simulink model "atrias_boom_nmSt_kinSw_v4"  (R2015a)
settings: Solver=ode23t  StartTime=0.0  StopTime=t_end  FixedStep=0.001  MaxStep=1e-3  RelTol=1e-3
InitFcn:
  | addpath('../common/')
  | colors
StartFcn:
  | tic
StopFcn:
  | %stopscript
values from neighbouring files (symbols this model uses):
  dt_a_dTrunk_boom = 5    [main_1_nmSt_kinSw.m]    (also in main_2_nmSt_kinSw_v2.m; main_3_nmSt_kinSw_v3.m; main_4_nmSt_kinSw_v4.m)
  dt_fade_boomCtrl = 2    [main_1_nmSt_kinSw.m]    (also in main_2_nmSt_kinSw_v2.m; main_3_nmSt_kinSw_v3.m; main_4_nmSt_kinSw_v4.m)
  initial_boom_yaw = 15*pi/180    (= 0.261799387799)    [main_2_nmSt_kinSw_v2.m]    (also in main_3_nmSt_kinSw_v3.m; main_4_nmSt_kinSw_v4.m)
  kd_boom_roll_Ctrl = 0    [main_1_nmSt_kinSw - Copy.m]    (also in main_1_nmSt_kinSw.m; main_2_nmSt_kinSw_v2.m; main_3_nmSt_kinSw_v3.m; main_4_nmSt_kinSw_v4.m)
  kd_boom_yaw_Ctrl = 0.1*kp_boom_yaw_Ctrl    (= 100000000)    [main_1_nmSt_kinSw - Copy.m]    (also in main_1_nmSt_kinSw.m = 1000000000; main_2_nmSt_kinSw_v2.m = 10000000; main_3_nmSt_kinSw_v3.m = 10000000; main_4_nmSt_kinSw_v4.m = 10000000)
  kd_motor = 0.90*2*sqrt(3.75*kp_motor)    [main_1_nmSt_kinSw - Copy.m]
  kinSw_alpha_start = 100*pi/180    (= 1.74532925199)    [main_1_nmSt_kinSw - Copy.m]    (also in main_1_nmSt_kinSw.m = 1.91986217719; main_2_nmSt_kinSw_v2.m = 1.83259571459; main_3_nmSt_kinSw_v3.m = 1.83259571459; main_4_nmSt_kinSw_v4.m = 1.83259571459)
  kinSw_alpha_tgt = 80*pi/180    (= 1.3962634016)    [main_1_nmSt_kinSw - Copy.m]    (also in main_1_nmSt_kinSw.m = 1.2217304764; main_2_nmSt_kinSw_v2.m = 1.2217304764; main_3_nmSt_kinSw_v3.m = 1.2217304764; main_4_nmSt_kinSw_v4.m = 1.2217304764)
  kinSw_t_start = 1.5    [main_1_nmSt_kinSw - Copy.m]    (also in main_1_nmSt_kinSw.m; main_2_nmSt_kinSw_v2.m = 0.5; main_3_nmSt_kinSw_v3.m = 0.5; main_4_nmSt_kinSw_v4.m = 0.5)
  kp_boom_roll_Ctrl = 0    [main_1_nmSt_kinSw - Copy.m]    (also in main_1_nmSt_kinSw.m; main_2_nmSt_kinSw_v2.m; main_3_nmSt_kinSw_v3.m; main_4_nmSt_kinSw_v4.m)
  kp_boom_yaw_Ctrl = 1e9    (= 1000000000)    [main_1_nmSt_kinSw - Copy.m]    (also in main_1_nmSt_kinSw.m = 10000000000; main_2_nmSt_kinSw_v2.m = 100000000; main_3_nmSt_kinSw_v3.m = 100000000; main_4_nmSt_kinSw_v4.m = 100000000)
  kp_motor = 3000    [main_1_nmSt_kinSw - Copy.m]
  max_back_bar_angle = 262.4*pi/180    (= 4.57974395723)    [main_1_nmSt_kinSw - Copy.m]
  max_front_bar_angle = 194.8*pi/180    (= 3.39990138288)    [main_1_nmSt_kinSw - Copy.m]
  min_back_bar_angle = 165.0*pi/180    (= 2.87979326579)    [main_1_nmSt_kinSw - Copy.m]
  min_front_bar_angle = 98.0*pi/180    (= 1.71042266695)    [main_1_nmSt_kinSw - Copy.m]
  poser_LLegAlp = (initial_l_leg_angle -pi/2)*180/pi    (= 105)    [main_2_nmSt_kinSw_v2.m]    (also in main_3_nmSt_kinSw_v3.m; main_4_nmSt_kinSw_v4.m)
  poser_LLegLen = initial_l_leg_length    (= 0.88)    [main_2_nmSt_kinSw_v2.m]    (also in main_3_nmSt_kinSw_v3.m; main_4_nmSt_kinSw_v4.m)
  poser_RLegAlp = (initial_r_leg_angle -pi/2)*180/pi    (= 75)    [main_2_nmSt_kinSw_v2.m]    (also in main_3_nmSt_kinSw_v3.m; main_4_nmSt_kinSw_v4.m)
  poser_RLegLen = initial_r_leg_length    (= 0.9)    [main_2_nmSt_kinSw_v2.m]    (also in main_3_nmSt_kinSw_v3.m; main_4_nmSt_kinSw_v4.m)
  tEnd_boomCtrl = t_end    (= 20)    [main_1_nmSt_kinSw - Copy.m]    (also in main_1_nmSt_kinSw.m = 3; main_2_nmSt_kinSw_v2.m = 7.5; main_3_nmSt_kinSw_v3.m = 7.5; main_4_nmSt_kinSw_v4.m = 7.5)
  tStart_boomCtrl = 1    [main_1_nmSt_kinSw - Copy.m]    (also in main_1_nmSt_kinSw.m = 0; main_2_nmSt_kinSw_v2.m = 0.5; main_3_nmSt_kinSw_v3.m = 0.5; main_4_nmSt_kinSw_v4.m = 0.5)
  tune_kinSw_alpha_start = kinSw_alpha_start*180/pi    (= 105)    [main_2_nmSt_kinSw_v2.m]    (also in main_3_nmSt_kinSw_v3.m; main_4_nmSt_kinSw_v4.m)
  tune_kinSw_alpha_tgt = kinSw_alpha_tgt*180/pi    (= 70)    [main_2_nmSt_kinSw_v2.m]    (also in main_3_nmSt_kinSw_v3.m; main_4_nmSt_kinSw_v4.m)
  tune_kinSw_gClr_tgt = kinSw_gClr    (= 0.15)    [main_4_nmSt_kinSw_v4.m]
  tune_kinSw_gH_tgt = kinSw_gH_tgt    (= -0.01)    [main_4_nmSt_kinSw_v4.m]
  tune_M1_G = St_FGain_VAS*FmaxVAS    [main_2_nmSt_kinSw_v2.m]    (also in main_3_nmSt_kinSw_v3.m; main_4_nmSt_kinSw_v4.m)
  tune_M3_0 = CtrlPar_theta0*180/pi    [main_2_nmSt_kinSw_v2.m]    (also in main_3_nmSt_kinSw_v3.m; main_4_nmSt_kinSw_v4.m)
  tune_M3_D = St_GainDTh_HFL    [main_2_nmSt_kinSw_v2.m]    (also in main_3_nmSt_kinSw_v3.m; main_4_nmSt_kinSw_v4.m)
  tune_M3_P = St_GainTh_HFL    [main_2_nmSt_kinSw_v2.m]    (also in main_3_nmSt_kinSw_v3.m; main_4_nmSt_kinSw_v4.m)
  tune_M4_G = 1    [main_3_nmSt_kinSw_v3.m]    (also in main_4_nmSt_kinSw_v4.m)
  v_dTrunk_boom = 1.3    [main_1_nmSt_kinSw.m]    (also in main_2_nmSt_kinSw_v2.m; main_3_nmSt_kinSw_v3.m; main_4_nmSt_kinSw_v4.m)
undefined symbols (not defined in the file or in its folder): A1_notch_f1, A2_notch_f1, A_lpf_dtau, A_lpf_velocity, ankle_stiffness, B1_lpf_dtau, B1_lpf_velocity, B1_notch_f1, B2_lpf_dtau, B2_lpf_velocity, B2_notch_f1, b_hmotor, b_leg_spring, b_rotor, base_color_d, boom_color_d, boom_mount_to_center_diagonal, breakaway_friction, c_jointstop, contactThr, coulomb_friction, d_com, delta_phi_max, delta_phi_max_buffer, delta_phi_max_dropoff, delta_phi_min, fblink_color_d, floor_color_d, FmaxBFSH, FmaxGLU, FmaxHAM, FmaxHFL, FmaxRF, FmaxVAS, foot_color_d, FPCtrlPar, friction_linear_zone, g, gain_nodes_sea_torque, HIP_MTR_MAX_CONT_TORQUE, HIP_MTR_MAX_TORQUE, hshaft_color_d, initial_boom_pitch, initial_boom_roll, initial_hip_roll, initial_winch_angle, j_motor, k_gn, k_gt, k_leg_spring, K_notch_f1, k_phi, k_sea, Kb_leg, kd_lateral, kd_shin_max, kd_shin_min, kd_splay_max, kd_splay_min, kd_thigh_max ... (+186)
libraries: sm_lib x210, nesl_utility x140, simulink x65, simulink_extras x32, fl_lib x16, mblibv1 x2, commnoisgen2 x1
(part 16 of 17)

== system atrias_boom_nmSt_kinSw_v4/Control/Behavior Control/Virtual Neuromuscular Control/Muscle Layer/VAS1/BE force-length relation ==
  note: Buffer Elasticity BE
  lce [lopt] : Inport
  Constant1 : Constant  Value=1-mtu_w
  Math Function : Math  Operator=square  SaturateOnIntegerOverflow=on
  Mux1 : Mux  Inputs=2
  Sum4 : Sum  Inputs=|+-  SaturateOnIntegerOverflow=on  InputSameDT=on  OutDataTypeStr=Inherit: Same as first input
  force above slack length : Fcn  Expr=u(2)*(u(1)<0)
  reference strain [lslack] : Constant  Value=mtu_w/2
  relative strain : Product  Inputs=*/
  fbe [Fmax] : Outport
  wires:
  lce [lopt]/1 -> Sum4/1
  Mux1/1 -> force above slack length/1
  force above slack length/1 -> fbe [Fmax]/1
  Math Function/1 -> Mux1/2
  relative strain/1 -> Math Function/1
  reference strain [lslack]/1 -> relative strain/2
  Sum4/1 -> relative strain/1, Mux1/1
  Constant1/1 -> Sum4/2

== system atrias_boom_nmSt_kinSw_v4/Control/Behavior Control/Virtual Neuromuscular Control/Muscle Layer/VAS1/CE force-length relation ==
  note: CE Force-Length Relationship
  lce [lopt] : Inport
  Abs : Abs
  Constant1 : Constant
  Constant2 : Constant  Value=3
  Gain : Gain  Gain=log(mtu_c)
  Math Function : Math  SaturateOnIntegerOverflow=on
  Math Function1 : Math  Operator=pow  SaturateOnIntegerOverflow=on
  Sum4 : Sum  Inputs=|+-  SaturateOnIntegerOverflow=on  InputSameDT=on  OutDataTypeStr=Inherit: Same as first input
  normalized position : Product  Inputs=*/
  relative width : Constant  Value=mtu_w
  fce [Fmax] : Outport
  wires:
  lce [lopt]/1 -> Sum4/1
  relative width/1 -> normalized position/2
  Constant1/1 -> Sum4/2
  Sum4/1 -> Abs/1
  Abs/1 -> normalized position/1
  normalized position/1 -> Math Function1/1
  Constant2/1 -> Math Function1/2
  Math Function1/1 -> Gain/1
  Gain/1 -> Math Function/1
  Math Function/1 -> fce [Fmax]/1

== system atrias_boom_nmSt_kinSw_v4/Control/Behavior Control/Virtual Neuromuscular Control/Muscle Layer/VAS1/CE inverse force-velocity relation ==
  note: CE Inverse Force-Velocity Relationship
  Fv[Fmax] : Inport
  1 : Product  Inputs=/*
  Constant{1,3..4,8} (4 alike) : Constant
  Constant2 : Constant  Value=mtu_N
  Constant5 : Constant  Value=mtu_N
  Curvature : Gain  Gain=mtu_K  SaturateOnIntegerOverflow=on  OutDataTypeStr=Inherit: Same as input  ParamDataTypeStr=Inherit: Same as input
  Curvature1 : Gain  Gain=7.56*mtu_K  SaturateOnIntegerOverflow=on  OutDataTypeStr=Inherit: Same as input  ParamDataTypeStr=Inherit: Same as input
  Mux : Mux  Inputs=2
  Mux1 : Mux  Inputs=3
  Mux2 : Mux  Inputs=3
  Slope : Gain  Gain=1e-2  SaturateOnIntegerOverflow=on  OutDataTypeStr=Inherit: Same as input  ParamDataTypeStr=Inherit: Same as input
  Sum1 : Sum  Inputs=|++  SaturateOnIntegerOverflow=on  InputSameDT=on  OutDataTypeStr=Inherit: Same as first input
  Sum2 : Sum  SaturateOnIntegerOverflow=on  InputSameDT=on  OutDataTypeStr=Inherit: Same as first input
  Sum3 : Sum  Inputs=++|  SaturateOnIntegerOverflow=on  InputSameDT=on  OutDataTypeStr=Inherit: Same as first input
  Sum4 : Sum  Inputs=|+-  SaturateOnIntegerOverflow=on  InputSameDT=on  OutDataTypeStr=Inherit: Same as first input
  Sum5 : Sum  Inputs=|-+  SaturateOnIntegerOverflow=on  InputSameDT=on  OutDataTypeStr=Inherit: Same as first input
  Sum6 : Sum  Inputs=-+|  SaturateOnIntegerOverflow=on  InputSameDT=on  OutDataTypeStr=Inherit: Same as first input
  Sum7 : Sum  Inputs=|++  SaturateOnIntegerOverflow=on  InputSameDT=on  OutDataTypeStr=Inherit: Same as first input
  Sum8 : Sum  Inputs=+-|  SaturateOnIntegerOverflow=on  InputSameDT=on  OutDataTypeStr=Inherit: Same as first input
  Sum9 : Sum  SaturateOnIntegerOverflow=on  InputSameDT=on  OutDataTypeStr=Inherit: Same as first input
  concentric branch : Fcn  Expr=u(1) * (u(2)<=1)
  excentric branch : Fcn  Expr=u(2) * (u(1)>1)*(u(1)<=u(3))
  excentric overshoot : Fcn  Expr=u(3) * (u(2)>u(1))
  v_concentric : Product  Inputs=*/
  v_excentric <N : Product  Inputs=*/
  v[vmax] : Outport
  wires:
  Curvature/1 -> Sum3/2
  Constant1/1 -> Sum4/2, Sum3/1
  Sum4/1 -> v_concentric/1
  Sum3/1 -> v_concentric/2
  1/1 -> Sum7/1, Curvature1/1
  Constant4/1 -> Sum7/2, Sum8/1
  Curvature1/1 -> Sum8/2
  Sum8/1 -> v_excentric <N/2
  Sum7/1 -> v_excentric <N/1
  v_concentric/1 -> Mux/1
  Fv[Fmax]/1 -> Sum4/1, Curvature/1, Sum6/2, Mux/2, Mux1/1, Mux2/2
  Sum9/1 -> v[vmax]/1
  Sum2/1 -> Sum9/2
  excentric overshoot/1 -> Sum2/2
  Slope/1 -> Sum1/1
  Constant8/1 -> Sum1/2
  Sum6/1 -> 1/2, Slope/1
  Constant2/1 -> Sum6/1, Sum5/2
  Sum5/1 -> 1/1
  Constant3/1 -> Sum5/1
  Mux/1 -> concentric branch/1
  Mux1/1 -> excentric branch/1
  v_excentric <N/1 -> Mux1/2
  Mux2/1 -> excentric overshoot/1
  concentric branch/1 -> Sum9/1
  excentric branch/1 -> Sum2/1
  Constant5/1 -> Mux1/3, Mux2/1
  Sum1/1 -> Mux2/3

== system atrias_boom_nmSt_kinSw_v4/Control/Behavior Control/Virtual Neuromuscular Control/Muscle Layer/VAS1/PE force-length relation ==
  note: Parallel Elasticity PE
  lce [lopt] : Inport
  Constant3 : Constant
  Math Function2 : Math  Operator=square  SaturateOnIntegerOverflow=on
  Mux : Mux  Inputs=2
  Sum1 : Sum  Inputs=|+-  SaturateOnIntegerOverflow=on  InputSameDT=on  OutDataTypeStr=Inherit: Same as first input
  force above slack length : Fcn  Expr=u(2) * (u(1)>1)
  reference strain [lopt] : Constant  Value=mtu_w
  relative strain : Product  Inputs=*/
  fpe [Fmax] : Outport
  wires:
  Mux/1 -> force above slack length/1
  lce [lopt]/1 -> Mux/1, Sum1/1
  Constant3/1 -> Sum1/2
  Sum1/1 -> relative strain/1
  reference strain [lopt]/1 -> relative strain/2
  relative strain/1 -> Math Function2/1
  Math Function2/1 -> Mux/2
  force above slack length/1 -> fpe [Fmax]/1

== system atrias_boom_nmSt_kinSw_v4/Control/Behavior Control/Virtual Neuromuscular Control/Muscle Layer/VAS1/SE force-length relation ==
  note: SE Force-Length Relationship
  lse [lslack] : Inport
  Constant1 : Constant
  Math Function : Math  Operator=square  SaturateOnIntegerOverflow=on
  Mux : Mux  Inputs=2
  Sum4 : Sum  Inputs=|+-  SaturateOnIntegerOverflow=on  InputSameDT=on  OutDataTypeStr=Inherit: Same as first input
  force above slack length : Fcn  Expr=u(2)*(u(1)>1)
  reference strain [lslack] : Constant  Value=mtu_eref
  relative strain : Product  Inputs=*/
  fse [Fmax] : Outport
  wires:
  Mux/1 -> force above slack length/1
  force above slack length/1 -> fse [Fmax]/1
  Math Function/1 -> Mux/2
  lse [lslack]/1 -> Mux/1, Sum4/1
  relative strain/1 -> Math Function/1
  reference strain [lslack]/1 -> relative strain/2
  Sum4/1 -> relative strain/1
  Constant1/1 -> Sum4/2

== system atrias_boom_nmSt_kinSw_v4/Control/Behavior Control/Virtual Neuromuscular Control/Torque Distribution/mech limit avoidance1/PD Joint Limit ==
  L Mechanical Limit Avoidance Torque : Subsystem
  L scale desired torque : Subsystem
  Mux1 : Mux
  Mux2 : Mux
  R Mechanical Limit Avoidance Torque : Subsystem
  R scale desired torque : Subsystem
  tau_pd_hip_knee [Nm]x4 : Outport
  des_trq_scale x4 : Outport  Port=2
  tag scope: L_scale_hip=global, L_scale_knee=global, Ltau_pd_hip=global, Ltau_pd_knee=global, R_scale_hip=global, R_scale_knee=global, Rtau_pd_hip=global, Rtau_pd_knee=global
  wires:
  L scale desired torque/2(scale_knee) -> [L_scale_knee]
  L scale desired torque/1(scale_hip) -> [L_scale_hip]
  [Lphi_shin] -> L scale desired torque/2(phi_shin [rad])
  [Lphi_thigh] -> L scale desired torque/1(phi_thigh [rad])
  R Mechanical Limit Avoidance Torque/1(tau_pd_hip [Nm]) -> [Rtau_pd_hip]
  L Mechanical Limit Avoidance Torque/2(tau_pd_knee [Nm]) -> [Ltau_pd_knee]
  L Mechanical Limit Avoidance Torque/1(tau_pd_hip [Nm]) -> [Ltau_pd_hip]
  R Mechanical Limit Avoidance Torque/2(tau_pd_knee [Nm]) -> [Rtau_pd_knee]
  Mux2/1 -> tau_pd_hip_knee [Nm]x4/1
  [Rtau_pd_hip] -> Mux2/1
  [Rtau_pd_knee] -> Mux2/2
  [Ltau_pd_hip] -> Mux2/3
  [Ltau_pd_knee] -> Mux2/4
  Mux1/1 -> des_trq_scale x4/1
  [R_scale_hip] -> Mux1/1
  [R_scale_knee] -> Mux1/2
  [L_scale_hip] -> Mux1/3
  [L_scale_knee] -> Mux1/4
  R scale desired torque/2(scale_knee) -> [R_scale_knee]
  R scale desired torque/1(scale_hip) -> [R_scale_hip]
  [Rphi_shin] -> R scale desired torque/2(phi_shin [rad])
  [Rphi_thigh] -> R scale desired torque/1(phi_thigh [rad])
  [Rdphi_shin] -> R Mechanical Limit Avoidance Torque/4(dphi_shin [rad/s])
  [Rdphi_thigh] -> R Mechanical Limit Avoidance Torque/3(dphi_thigh [rad/s])
  [Rphi_shin] -> R Mechanical Limit Avoidance Torque/2(phi_shin [rad])
  [Rphi_thigh] -> R Mechanical Limit Avoidance Torque/1(phi_thigh [rad])
  [Ldphi_shin] -> L Mechanical Limit Avoidance Torque/4(dphi_shin [rad/s])
  [Ldphi_thigh] -> L Mechanical Limit Avoidance Torque/3(dphi_thigh [rad/s])
  [Lphi_shin] -> L Mechanical Limit Avoidance Torque/2(phi_shin [rad])
  [Lphi_thigh] -> L Mechanical Limit Avoidance Torque/1(phi_thigh [rad])

== system atrias_boom_nmSt_kinSw_v4/Control/Behavior Control/Virtual Neuromuscular Control/Torque Distribution/mech limit avoidance1/PD Joint Limit1 ==
  Demux : Demux
  Lechanical Limit Avoidance Torques : Subsystem
  Mux1 : Mux
  R Mechanical Limit Avoidance Torque : Subsystem
  R scale desired torque : Subsystem
  R scale desired torque1 : Subsystem
  to hip_knee : MATLAB Function  TreatAsAtomicUnit=on
  tau_pd_hip_knee [Nm]x4 : Outport
  des_trq_scale x4 : Outport  Port=2
  tag scope: L_scale_hip=global, L_scale_knee=global, Ltau_pd_back=global, Ltau_pd_front=global, Ltau_pd_hip=global, Ltau_pd_knee=global, R_scale_hip=global, R_scale_knee=global, Rtau_pd_back=global, Rtau_pd_front=global, Rtau_pd_hip=global, Rtau_pd_knee=global
  wires:
  [Lphi_thigh] -> Lechanical Limit Avoidance Torques/1(phi_thigh [rad])
  [Lphi_shin] -> Lechanical Limit Avoidance Torques/2(phi_shin [rad])
  [Ldphi_thigh] -> Lechanical Limit Avoidance Torques/3(dphi_thigh [rad/s])
  [Ldphi_shin] -> Lechanical Limit Avoidance Torques/4(dphi_shin [rad/s])
  Lechanical Limit Avoidance Torques/1(tau_pd_back [Nm]) -> [Ltau_pd_back]
  Lechanical Limit Avoidance Torques/2(tau_pd_front [Nm]) -> [Ltau_pd_front]
  [Rphi_thigh] -> R Mechanical Limit Avoidance Torque/1(phi_thigh [rad])
  [Rphi_shin] -> R Mechanical Limit Avoidance Torque/2(phi_shin [rad])
  [Rdphi_thigh] -> R Mechanical Limit Avoidance Torque/3(dphi_thigh [rad/s])
  [Rdphi_shin] -> R Mechanical Limit Avoidance Torque/4(dphi_shin [rad/s])
  R Mechanical Limit Avoidance Torque/1(tau_pd_back [Nm]) -> [Rtau_pd_back]
  R Mechanical Limit Avoidance Torque/2(tau_pd_front [Nm]) -> [Rtau_pd_front]
  [Rphi_thigh] -> R scale desired torque/1(phi_thigh [rad])
  [Rphi_shin] -> R scale desired torque/2(phi_shin [rad])
  R scale desired torque/1(scale_hip) -> [R_scale_hip]
  R scale desired torque/2(scale_knee) -> [R_scale_knee]
  [k_R] -> to hip_knee/5(kR)
  [k_L] -> to hip_knee/6(kL)
  [Ltau_pd_front] -> to hip_knee/4(Ltau_front)
  [Ltau_pd_back] -> to hip_knee/3(Ltau_back)
  [Rtau_pd_front] -> to hip_knee/2(Rtau_front)
  [Rtau_pd_back] -> to hip_knee/1(Rtau_back)
  to hip_knee/1(tau_pd_hip_knee) -> tau_pd_hip_knee [Nm]x4/1, Demux/1
  [k_R] -> R scale desired torque/3(k)
  [Lphi_thigh] -> R scale desired torque1/1(phi_thigh [rad])
  [Lphi_shin] -> R scale desired torque1/2(phi_shin [rad])
  R scale desired torque1/1(scale_hip) -> [L_scale_hip]
  R scale desired torque1/2(scale_knee) -> [L_scale_knee]
  [k_L] -> R scale desired torque1/3(k)
  [L_scale_knee] -> Mux1/4
  [L_scale_hip] -> Mux1/3
  [R_scale_knee] -> Mux1/2
  [R_scale_hip] -> Mux1/1
  Mux1/1 -> des_trq_scale x4/1
  Demux/1 -> [Rtau_pd_hip]
  Demux/2 -> [Rtau_pd_knee]
  Demux/3 -> [Ltau_pd_hip]
  Demux/4 -> [Ltau_pd_knee]

== system atrias_boom_nmSt_kinSw_v4/Mechanical System Layer/Ground Contact Models/L Back Ground Contact/3D Contact/Kinetic Friction Model/Vector Norm ==
  vec : Inport
  Sqrt : Sqrt  OutputSignalType=real  AlgorithmType=Newton-Raphson  SaturateOnIntegerOverflow=on
  Squares : Math  Operator=square  OutputSignalType=real  SaturateOnIntegerOverflow=on
  Sum of Elements : Sum  Inputs=+
  norm : Outport
  wires:
  vec/1 -> Squares/1
  Sqrt/1 -> norm/1
  Sum of Elements/1 -> Sqrt/1
  Squares/1 -> Sum of Elements/1

== system atrias_boom_nmSt_kinSw_v4/Mechanical System Layer/Ground Contact Models/L Back Ground Contact/3D Contact/Static Friction Model/Vector Norm ==
  vec : Inport
  Sqrt : Sqrt  OutputSignalType=real  AlgorithmType=Newton-Raphson  SaturateOnIntegerOverflow=on
  Squares : Math  Operator=square  OutputSignalType=real  SaturateOnIntegerOverflow=on
  Sum of Elements : Sum  Inputs=+
  norm : Outport
  wires:
  vec/1 -> Squares/1
  Sqrt/1 -> norm/1
  Sum of Elements/1 -> Sqrt/1
  Squares/1 -> Sum of Elements/1

== system atrias_boom_nmSt_kinSw_v4/Mechanical System Layer/Ground Contact Models/L Front Ground Contact/3D Contact/Kinetic Friction Model/Vector Norm ==
  vec : Inport
  Sqrt : Sqrt  OutputSignalType=real  AlgorithmType=Newton-Raphson  SaturateOnIntegerOverflow=on
  Squares : Math  Operator=square  OutputSignalType=real  SaturateOnIntegerOverflow=on
  Sum of Elements : Sum  Inputs=+
  norm : Outport
  wires:
  vec/1 -> Squares/1
  Sqrt/1 -> norm/1
  Sum of Elements/1 -> Sqrt/1
  Squares/1 -> Sum of Elements/1

== system atrias_boom_nmSt_kinSw_v4/Mechanical System Layer/Ground Contact Models/L Front Ground Contact/3D Contact/Static Friction Model/Vector Norm ==
  vec : Inport
  Sqrt : Sqrt  OutputSignalType=real  AlgorithmType=Newton-Raphson  SaturateOnIntegerOverflow=on
  Squares : Math  Operator=square  OutputSignalType=real  SaturateOnIntegerOverflow=on
  Sum of Elements : Sum  Inputs=+
  norm : Outport
  wires:
  vec/1 -> Squares/1
  Sqrt/1 -> norm/1
  Sum of Elements/1 -> Sqrt/1
  Squares/1 -> Sum of Elements/1

== system atrias_boom_nmSt_kinSw_v4/Mechanical System Layer/Ground Contact Models/R Back Ground Contact/3D Contact/Kinetic Friction Model/Vector Norm ==
  vec : Inport
  Sqrt : Sqrt  OutputSignalType=real  AlgorithmType=Newton-Raphson  SaturateOnIntegerOverflow=on
  Squares : Math  Operator=square  OutputSignalType=real  SaturateOnIntegerOverflow=on
  Sum of Elements : Sum  Inputs=+
  norm : Outport
  wires:
  vec/1 -> Squares/1
  Sqrt/1 -> norm/1
  Sum of Elements/1 -> Sqrt/1
  Squares/1 -> Sum of Elements/1

== system atrias_boom_nmSt_kinSw_v4/Mechanical System Layer/Ground Contact Models/R Back Ground Contact/3D Contact/Static Friction Model/Vector Norm ==
  vec : Inport
  Sqrt : Sqrt  OutputSignalType=real  AlgorithmType=Newton-Raphson  SaturateOnIntegerOverflow=on
  Squares : Math  Operator=square  OutputSignalType=real  SaturateOnIntegerOverflow=on
  Sum of Elements : Sum  Inputs=+
  norm : Outport
  wires:
  vec/1 -> Squares/1
  Sqrt/1 -> norm/1
  Sum of Elements/1 -> Sqrt/1
  Squares/1 -> Sum of Elements/1

== system atrias_boom_nmSt_kinSw_v4/Mechanical System Layer/Ground Contact Models/R Front Ground Contact/3D Contact/Kinetic Friction Model/Vector Norm ==
  vec : Inport
  Sqrt : Sqrt  OutputSignalType=real  AlgorithmType=Newton-Raphson  SaturateOnIntegerOverflow=on
  Squares : Math  Operator=square  OutputSignalType=real  SaturateOnIntegerOverflow=on
  Sum of Elements : Sum  Inputs=+
  norm : Outport
  wires:
  vec/1 -> Squares/1
  Sqrt/1 -> norm/1
  Sum of Elements/1 -> Sqrt/1
  Squares/1 -> Sum of Elements/1

== system atrias_boom_nmSt_kinSw_v4/Mechanical System Layer/Ground Contact Models/R Front Ground Contact/3D Contact/Static Friction Model/Vector Norm ==
  vec : Inport
  Sqrt : Sqrt  OutputSignalType=real  AlgorithmType=Newton-Raphson  SaturateOnIntegerOverflow=on
  Squares : Math  Operator=square  OutputSignalType=real  SaturateOnIntegerOverflow=on
  Sum of Elements : Sum  Inputs=+
  norm : Outport
  wires:
  vec/1 -> Squares/1
  Sqrt/1 -> norm/1
  Sum of Elements/1 -> Sqrt/1
  Squares/1 -> Sum of Elements/1

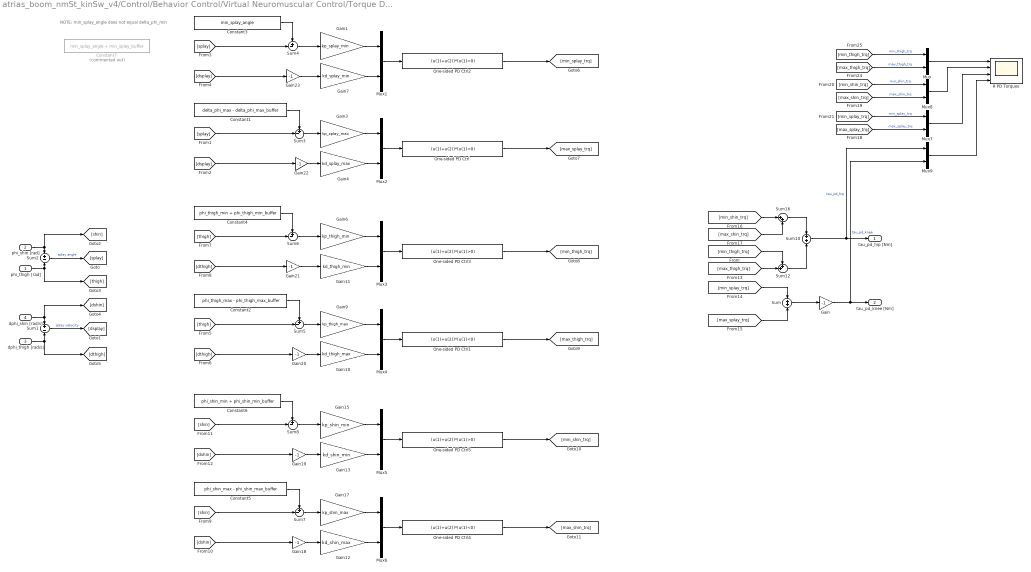
== system atrias_boom_nmSt_kinSw_v4/Control/Behavior Control/Virtual Neuromuscular Control/Torque Distribution/mech limit avoidance1/PD Joint Limit/L Mechanical Limit Avoidance Torque ==
  note: NOTE: min_splay_angle does not equal delta_phi_min
  phi_thigh [rad] : Inport
  phi_shin [rad] : Inport  Port=2
  dphi_thigh [rad/s] : Inport  Port=3
  dphi_shin [rad/s] : Inport  Port=4
  Constant1 : Constant  Value=delta_phi_max - delta_phi_max_buffer
  Constant2 : Constant  Value=phi_thigh_max - phi_thigh_max_buffer
  Constant3 : Constant  Value=min_splay_angle
  Constant4 : Constant  Value=phi_thigh_min + phi_thigh_min_buffer
  Constant5 : Constant  Value=phi_shin_max - phi_shin_max_buffer
  Constant6 : Constant  Value=phi_shin_min + phi_shin_min_buffer
  Constant7 : Constant  Commented=on  Value=min_splay_angle + min_splay_buffer
  Gain{,18..23} (7 alike) : Gain  Gain=-1
  Gain1 : Gain  Gain=kp_splay_min
  Gain10 : Gain  Gain=kd_thigh_max
  Gain11 : Gain  Gain=kd_thigh_min
  Gain12 : Gain  Gain=kd_shin_max
  Gain13 : Gain  Gain=kd_shin_min
  Gain15 : Gain  Gain=kp_shin_min
  Gain17 : Gain  Gain=kp_shin_max
  Gain3 : Gain  Gain=kp_splay_max
  Gain4 : Gain  Gain=kd_splay_max
  Gain6 : Gain  Gain=kp_thigh_min
  Gain7 : Gain  Gain=kd_splay_min
  Gain9 : Gain  Gain=kp_thigh_max
  Mux{,1..9} (10 alike) : Mux  Inputs=2
  One-sided PD Ctrl : Fcn  Expr=(u(1)+u(2))*(u(1)<0)
  One-sided PD Ctrl1 : Fcn  Expr=(u(1)+u(2))*(u(1)<0)
  One-sided PD Ctrl2 : Fcn  Expr=(u(1)+u(2))*(u(1)>0)
  One-sided PD Ctrl3 : Fcn  Expr=(u(1)+u(2))*(u(1)>0)
  One-sided PD Ctrl4 : Fcn  Expr=(u(1)+u(2))*(u(1)<0)
  One-sided PD Ctrl5 : Fcn  Expr=(u(1)+u(2))*(u(1)>0)
  R PD Torques : Scope  NumInputPorts=4
      settings: ShowLegends=on  TimeRange=2.5  YMin=-100~-5e+07~-1e+07~-5  YMax=100~1e+07~5e+07~5  SaveName=ScopeData5
  Sum : Sum
  Sum1 : Sum  Inputs=+-
  Sum10 : Sum
  Sum12 : Sum  Inputs=++|
  Sum16 : Sum  Inputs=|++
  Sum2 : Sum  Inputs=+-
  Sum{3..8} (6 alike) : Sum  Inputs=+-|
  tau_pd_hip [Nm] : Outport
  tau_pd_knee [Nm] : Outport  Port=2
  wires:
  One-sided PD Ctrl4/1 -> [max_shin_trq]
  One-sided PD Ctrl5/1 -> [min_shin_trq]
  One-sided PD Ctrl1/1 -> [max_thigh_trq]
  One-sided PD Ctrl3/1 -> [min_thigh_trq]
  One-sided PD Ctrl/1 -> [max_splay_trq]
  Gain23/1 -> Gain7/1
  Gain22/1 -> Gain4/1
  Gain21/1 -> Gain11/1
  Gain20/1 -> Gain10/1
  Gain19/1 -> Gain13/1
  Gain18/1 -> Gain12/1
  [max_splay_trq] -> Mux7/2  "max_splay_trq"
  [min_splay_trq] -> Mux7/1  "min_splay_trq"
  Mux7/1 -> R PD Torques/3
  Mux8/1 -> R PD Torques/2
  [max_shin_trq] -> Mux8/2  "max_shin_trq"
  [min_shin_trq] -> Mux8/1  "min_shin_trq"
  Mux/1 -> R PD Torques/1
  [max_thigh_trq] -> Mux/2  "max_thigh_trq"
  [min_thigh_trq] -> Mux/1  "min_thigh_trq"
  One-sided PD Ctrl2/1 -> [min_splay_trq]
  Mux6/1 -> One-sided PD Ctrl4/1
  Constant5/1 -> Sum7/1
  Sum7/1 -> Gain17/1
  Gain17/1 -> Mux6/1
  Gain12/1 -> Mux6/2
  [shin] -> Sum7/2
  [dshin] -> Gain18/1
  Mux5/1 -> One-sided PD Ctrl5/1
  Constant6/1 -> Sum8/1
  Sum8/1 -> Gain15/1
  Gain15/1 -> Mux5/1
  Gain13/1 -> Mux5/2
  [shin] -> Sum8/2
  [dshin] -> Gain19/1
  Mux4/1 -> One-sided PD Ctrl1/1
  Constant2/1 -> Sum5/1
  Sum5/1 -> Gain9/1
  Gain9/1 -> Mux4/1
  Gain10/1 -> Mux4/2
  [thigh] -> Sum5/2
  [dthigh] -> Gain20/1
  Mux3/1 -> One-sided PD Ctrl3/1
  Constant4/1 -> Sum6/1
  Sum6/1 -> Gain6/1
  Gain6/1 -> Mux3/1
  Gain11/1 -> Mux3/2
  [thigh] -> Sum6/2
  [dthigh] -> Gain21/1
  Mux2/1 -> One-sided PD Ctrl/1
  Constant1/1 -> Sum3/1
  Sum3/1 -> Gain3/1
  Gain3/1 -> Mux2/1
  Gain4/1 -> Mux2/2
  [splay] -> Sum3/2
  [dsplay] -> Gain22/1
  Mux1/1 -> One-sided PD Ctrl2/1
  Constant3/1 -> Sum4/1
  Sum4/1 -> Gain1/1
  Gain1/1 -> Mux1/1
  Gain7/1 -> Mux1/2
  [splay] -> Sum4/2
  [dsplay] -> Gain23/1
  Sum1/1 -> [dsplay]  "splay velocity"
  Sum2/1 -> [splay]  "splay angle"
  phi_thigh [rad]/1 -> Sum2/2, [thigh]
  phi_shin [rad]/1 -> Sum2/1, [shin]
  dphi_thigh [rad/s]/1 -> Sum1/2, [dthigh]
  dphi_shin [rad/s]/1 -> Sum1/1, [dshin]
  [min_splay_trq] -> Sum/1
  [max_splay_trq] -> Sum/2
  Sum/1 -> Gain/1
  Gain/1 -> Mux9/2, tau_pd_knee [Nm]/1  "tau_pd_knee"
  [max_thigh_trq] -> Sum12/2
  [min_thigh_trq] -> Sum12/1
  [min_shin_trq] -> Sum16/1
  [max_shin_trq] -> Sum16/2
  Sum16/1 -> Sum10/1
  Sum12/1 -> Sum10/2
  Sum10/1 -> Mux9/1, tau_pd_hip [Nm]/1  "tau_pd_hip"
  Mux9/1 -> R PD Torques/4

== system atrias_boom_nmSt_kinSw_v4/Control/Behavior Control/Virtual Neuromuscular Control/Torque Distribution/mech limit avoidance1/PD Joint Limit/L scale desired torque ==
  note: NOTE: min_splay_angle does not equal delta_phi_min
  phi_thigh [rad] : Inport
  phi_shin [rad] : Inport  Port=2
  Constant : Constant
  Constant1 : Constant  Value=delta_phi_max - delta_phi_max_buffer
  Constant10 : Constant  Value=phi_thigh_max_buffer
  Constant11 : Constant  Value=phi_shin_min_buffer
  Constant12 : Constant  Value=phi_shin_max_buffer
  Constant13 : Constant
  Constant2 : Constant  Value=phi_thigh_max - phi_thigh_max_buffer
  Constant3 : Constant  Value=min_splay_angle
  Constant4 : Constant  Value=phi_thigh_min + phi_thigh_min_buffer
  Constant5 : Constant  Value=phi_shin_max - phi_shin_max_buffer
  Constant6 : Constant  Value=phi_shin_min + phi_shin_min_buffer
  Constant7 : Constant  Value=min_splay_angle - delta_phi_min
  Constant8 : Constant  Value=delta_phi_max_buffer
  Constant9 : Constant  Value=phi_thigh_min_buffer
  Divide{,1..5} (6 alike) : Product  Inputs=/*
  Gain : Gain  Gain=-1
  Gain1 : Gain  Gain=-1
  Gain2 : Gain  Gain=-1
  L scale hip/knee : Scope  NumInputPorts=4
      settings: ShowLegends=on  TimeRange=2.5  YMin=-100~-5e+07~-1e+07~-5  YMax=100~1e+07~5e+07~5  SaveName=ScopeData5
  Mux{,3,7..8} (4 alike) : Mux  Inputs=2
  Sum : Sum  Inputs=|+-
  Sum1 : Sum  Inputs=-+|
  Sum2 : Sum  Inputs=+-
  Sum{3..8} (6 alike) : Sum  Inputs=+-|
  [0,1]{,1..5} (6 alike) : Saturate  UpperLimit=1  LowerLimit=0
  max : MinMax  Function=max  Inputs=2
  max1 : MinMax  Function=max  Inputs=4
  scale_hip : Outport
  scale_knee : Outport  Port=2
  wires:
  max/1 -> Sum1/1
  max1/1 -> Sum/2
  phi_shin [rad]/1 -> [shin], Sum2/1
  phi_thigh [rad]/1 -> [thigh], Sum2/2
  Sum2/1 -> [splay]  "splay angle"
  [splay] -> Sum4/2
  Constant3/1 -> Sum4/1
  [splay] -> Sum3/2
  Constant1/1 -> Sum3/1
  [thigh] -> Sum6/2
  Constant4/1 -> Sum6/1
  [thigh] -> Sum5/2
  Constant2/1 -> Sum5/1
  [shin] -> Sum8/2
  Constant6/1 -> Sum8/1
  [shin] -> Sum7/2
  Constant5/1 -> Sum7/1
  [min_thigh_scale] -> Mux/1  "min_thigh_scale"
  [max_thigh_scale] -> Mux/2  "max_thigh_scale"
  Mux/1 -> L scale hip/knee/1
  [min_shin_scale] -> Mux8/1  "min_shin_scale"
  [max_shin_scale] -> Mux8/2  "max_shin_scale"
  Mux8/1 -> L scale hip/knee/2
  Mux7/1 -> L scale hip/knee/3
  [min_splay_scale] -> Mux7/1  "min_splay_scale"
  [max_splay_scale] -> Mux7/2  "max_splay_scale"
  Sum/1 -> Mux3/1, scale_hip/1
  Constant/1 -> Sum/1
  Constant7/1 -> Divide/1
  Sum4/1 -> Divide/2
  Divide/1 -> "[0,1]"/1
  "[0,1]"/1 -> [min_splay_scale]
  Divide1/1 -> "[0,1]1"/1
  "[0,1]1"/1 -> [max_splay_scale]
  Sum3/1 -> Gain/1
  Constant8/1 -> Divide1/1
  Gain/1 -> Divide1/2
  Divide2/1 -> "[0,1]2"/1
  "[0,1]2"/1 -> [min_thigh_scale]
  Sum6/1 -> Divide2/2
  Constant9/1 -> Divide2/1
  Divide3/1 -> "[0,1]3"/1
  "[0,1]3"/1 -> [max_thigh_scale]
  Gain1/1 -> Divide3/2
  Sum5/1 -> Gain1/1
  Constant10/1 -> Divide3/1
  Divide4/1 -> "[0,1]4"/1
  "[0,1]4"/1 -> [min_shin_scale]
  Sum8/1 -> Divide4/2
  Constant11/1 -> Divide4/1
  Divide5/1 -> "[0,1]5"/1
  "[0,1]5"/1 -> [max_shin_scale]
  Sum7/1 -> Gain2/1
  Constant12/1 -> Divide5/1
  Gain2/1 -> Divide5/2
  Constant13/1 -> Sum1/2
  Sum1/1 -> Mux3/2, scale_knee/1
  Mux3/1 -> L scale hip/knee/4
  [min_splay_scale] -> max/1
  [max_splay_scale] -> max/2
  [max_thigh_scale] -> max1/4
  [min_thigh_scale] -> max1/3
  [max_shin_scale] -> max1/2
  [min_shin_scale] -> max1/1

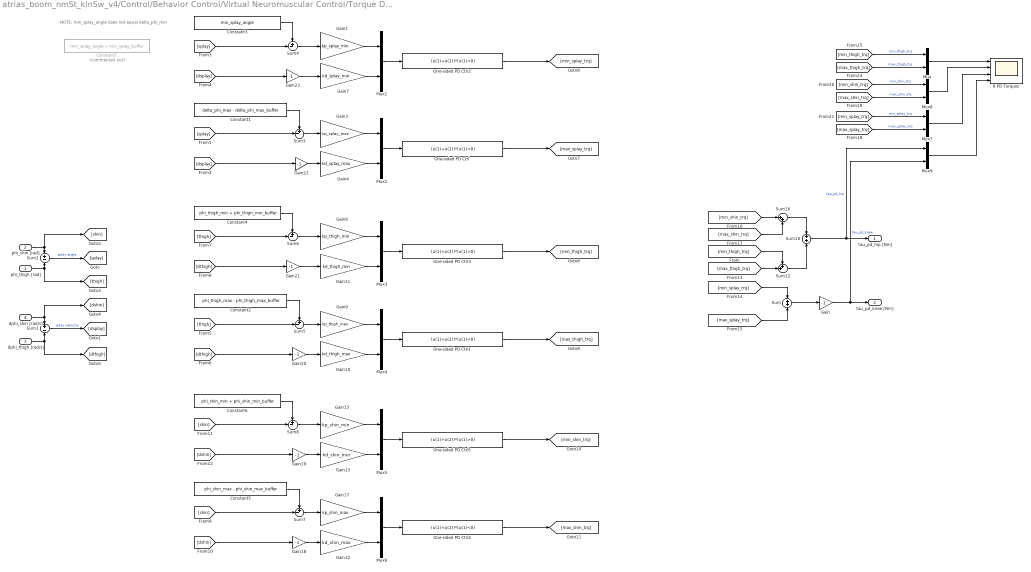
== system atrias_boom_nmSt_kinSw_v4/Control/Behavior Control/Virtual Neuromuscular Control/Torque Distribution/mech limit avoidance1/PD Joint Limit/R Mechanical Limit Avoidance Torque ==
  note: NOTE: min_splay_angle does not equal delta_phi_min
  phi_thigh [rad] : Inport
  phi_shin [rad] : Inport  Port=2
  dphi_thigh [rad/s] : Inport  Port=3
  dphi_shin [rad/s] : Inport  Port=4
  Constant1 : Constant  Value=delta_phi_max - delta_phi_max_buffer
  Constant2 : Constant  Value=phi_thigh_max - phi_thigh_max_buffer
  Constant3 : Constant  Value=min_splay_angle
  Constant4 : Constant  Value=phi_thigh_min + phi_thigh_min_buffer
  Constant5 : Constant  Value=phi_shin_max - phi_shin_max_buffer
  Constant6 : Constant  Value=phi_shin_min + phi_shin_min_buffer
  Constant7 : Constant  Commented=on  Value=min_splay_angle + min_splay_buffer
  Gain{,18..23} (7 alike) : Gain  Gain=-1
  Gain1 : Gain  Gain=kp_splay_min
  Gain10 : Gain  Gain=kd_thigh_max
  Gain11 : Gain  Gain=kd_thigh_min
  Gain12 : Gain  Gain=kd_shin_max
  Gain13 : Gain  Gain=kd_shin_min
  Gain15 : Gain  Gain=kp_shin_min
  Gain17 : Gain  Gain=kp_shin_max
  Gain3 : Gain  Gain=kp_splay_max
  Gain4 : Gain  Gain=kd_splay_max
  Gain6 : Gain  Gain=kp_thigh_min
  Gain7 : Gain  Gain=kd_splay_min
  Gain9 : Gain  Gain=kp_thigh_max
  Mux{,1..9} (10 alike) : Mux  Inputs=2
  One-sided PD Ctrl : Fcn  Expr=(u(1)+u(2))*(u(1)<0)
  One-sided PD Ctrl1 : Fcn  Expr=(u(1)+u(2))*(u(1)<0)
  One-sided PD Ctrl2 : Fcn  Expr=(u(1)+u(2))*(u(1)>0)
  One-sided PD Ctrl3 : Fcn  Expr=(u(1)+u(2))*(u(1)>0)
  One-sided PD Ctrl4 : Fcn  Expr=(u(1)+u(2))*(u(1)<0)
  One-sided PD Ctrl5 : Fcn  Expr=(u(1)+u(2))*(u(1)>0)
  R PD Torques : Scope  NumInputPorts=4
      settings: ShowLegends=on  TimeRange=2.5  YMin=-100~-5e+07~-1e+07~-5  YMax=100~1e+07~5e+07~5  SaveName=ScopeData5
  Sum : Sum
  Sum1 : Sum  Inputs=+-
  Sum10 : Sum
  Sum12 : Sum  Inputs=++|
  Sum16 : Sum  Inputs=|++
  Sum2 : Sum  Inputs=+-
  Sum{3..8} (6 alike) : Sum  Inputs=+-|
  tau_pd_hip [Nm] : Outport
  tau_pd_knee [Nm] : Outport  Port=2
  wires:
  Mux9/1 -> R PD Torques/4
  Sum10/1 -> tau_pd_hip [Nm]/1, Mux9/1  "tau_pd_hip"
  Sum12/1 -> Sum10/2
  Sum16/1 -> Sum10/1
  [max_shin_trq] -> Sum16/2
  [min_shin_trq] -> Sum16/1
  [min_thigh_trq] -> Sum12/1
  [max_thigh_trq] -> Sum12/2
  Gain/1 -> tau_pd_knee [Nm]/1, Mux9/2  "tau_pd_knee"
  Sum/1 -> Gain/1
  [max_splay_trq] -> Sum/2
  [min_splay_trq] -> Sum/1
  dphi_shin [rad/s]/1 -> [dshin], Sum1/1
  dphi_thigh [rad/s]/1 -> [dthigh], Sum1/2
  phi_shin [rad]/1 -> [shin], Sum2/1
  phi_thigh [rad]/1 -> [thigh], Sum2/2
  Sum2/1 -> [splay]  "splay angle"
  Sum1/1 -> [dsplay]  "splay velocity"
  [dsplay] -> Gain23/1
  [splay] -> Sum4/2
  Gain7/1 -> Mux1/2
  Gain1/1 -> Mux1/1
  Sum4/1 -> Gain1/1
  Constant3/1 -> Sum4/1
  Mux1/1 -> One-sided PD Ctrl2/1
  [dsplay] -> Gain22/1
  [splay] -> Sum3/2
  Gain4/1 -> Mux2/2
  Gain3/1 -> Mux2/1
  Sum3/1 -> Gain3/1
  Constant1/1 -> Sum3/1
  Mux2/1 -> One-sided PD Ctrl/1
  [dthigh] -> Gain21/1
  [thigh] -> Sum6/2
  Gain11/1 -> Mux3/2
  Gain6/1 -> Mux3/1
  Sum6/1 -> Gain6/1
  Constant4/1 -> Sum6/1
  Mux3/1 -> One-sided PD Ctrl3/1
  [dthigh] -> Gain20/1
  [thigh] -> Sum5/2
  Gain10/1 -> Mux4/2
  Gain9/1 -> Mux4/1
  Sum5/1 -> Gain9/1
  Constant2/1 -> Sum5/1
  Mux4/1 -> One-sided PD Ctrl1/1
  [dshin] -> Gain19/1
  [shin] -> Sum8/2
  Gain13/1 -> Mux5/2
  Gain15/1 -> Mux5/1
  Sum8/1 -> Gain15/1
  Constant6/1 -> Sum8/1
  Mux5/1 -> One-sided PD Ctrl5/1
  [dshin] -> Gain18/1
  [shin] -> Sum7/2
  Gain12/1 -> Mux6/2
  Gain17/1 -> Mux6/1
  Sum7/1 -> Gain17/1
  Constant5/1 -> Sum7/1
  Mux6/1 -> One-sided PD Ctrl4/1
  One-sided PD Ctrl2/1 -> [min_splay_trq]
  [min_thigh_trq] -> Mux/1  "min_thigh_trq"
  [max_thigh_trq] -> Mux/2  "max_thigh_trq"
  Mux/1 -> R PD Torques/1
  [min_shin_trq] -> Mux8/1  "min_shin_trq"
  [max_shin_trq] -> Mux8/2  "max_shin_trq"
  Mux8/1 -> R PD Torques/2
  Mux7/1 -> R PD Torques/3
  [min_splay_trq] -> Mux7/1  "min_splay_trq"
  [max_splay_trq] -> Mux7/2  "max_splay_trq"
  Gain18/1 -> Gain12/1
  Gain19/1 -> Gain13/1
  Gain20/1 -> Gain10/1
  Gain21/1 -> Gain11/1
  Gain22/1 -> Gain4/1
  Gain23/1 -> Gain7/1
  One-sided PD Ctrl/1 -> [max_splay_trq]
  One-sided PD Ctrl3/1 -> [min_thigh_trq]
  One-sided PD Ctrl1/1 -> [max_thigh_trq]
  One-sided PD Ctrl5/1 -> [min_shin_trq]
  One-sided PD Ctrl4/1 -> [max_shin_trq]

== system atrias_boom_nmSt_kinSw_v4/Control/Behavior Control/Virtual Neuromuscular Control/Torque Distribution/mech limit avoidance1/PD Joint Limit/R scale desired torque ==
  note: NOTE: min_splay_angle does not equal delta_phi_min
  phi_thigh [rad] : Inport
  phi_shin [rad] : Inport  Port=2
  Constant : Constant
  Constant1 : Constant  Value=delta_phi_max - delta_phi_max_buffer
  Constant10 : Constant  Value=phi_thigh_max_buffer
  Constant11 : Constant  Value=phi_shin_min_buffer
  Constant12 : Constant  Value=phi_shin_max_buffer
  Constant13 : Constant
  Constant2 : Constant  Value=phi_thigh_max - phi_thigh_max_buffer
  Constant3 : Constant  Value=min_splay_angle
  Constant4 : Constant  Value=phi_thigh_min + phi_thigh_min_buffer
  Constant5 : Constant  Value=phi_shin_max - phi_shin_max_buffer
  Constant6 : Constant  Value=phi_shin_min + phi_shin_min_buffer
  Constant7 : Constant  Value=min_splay_angle - delta_phi_min
  Constant8 : Constant  Value=delta_phi_max_buffer
  Constant9 : Constant  Value=phi_thigh_min_buffer
  Divide{,1..5} (6 alike) : Product  Inputs=/*
  Gain : Gain  Gain=-1
  Gain1 : Gain  Gain=-1
  Gain2 : Gain  Gain=-1
  Mux{,3,7..8} (4 alike) : Mux  Inputs=2
  R scale hip/knee : Scope  NumInputPorts=4
      settings: ShowLegends=on  TimeRange=0.8951752322126555  YMin=0~-1~0~0  YMax=1~1~1~1  SaveName=ScopeData5
  Sum : Sum  Inputs=|+-
  Sum1 : Sum  Inputs=-+|
  Sum2 : Sum  Inputs=+-
  Sum{3..8} (6 alike) : Sum  Inputs=+-|
  [0,1]{,1..5} (6 alike) : Saturate  UpperLimit=1  LowerLimit=0
  max : MinMax  Function=max  Inputs=2
  max1 : MinMax  Function=max  Inputs=4
  scale_hip : Outport
  scale_knee : Outport  Port=2
  wires:
  max/1 -> Sum1/1
  max1/1 -> Sum/2
  [min_shin_scale] -> max1/1
  [max_shin_scale] -> max1/2
  [min_thigh_scale] -> max1/3
  [max_thigh_scale] -> max1/4
  [max_splay_scale] -> max/2
  [min_splay_scale] -> max/1
  Mux3/1 -> R scale hip/knee/4
  Sum1/1 -> scale_knee/1, Mux3/2
  Constant13/1 -> Sum1/2
  Gain2/1 -> Divide5/2
  Constant12/1 -> Divide5/1
  Sum7/1 -> Gain2/1
  "[0,1]5"/1 -> [max_shin_scale]
  Divide5/1 -> "[0,1]5"/1
  Constant11/1 -> Divide4/1
  Sum8/1 -> Divide4/2
  "[0,1]4"/1 -> [min_shin_scale]
  Divide4/1 -> "[0,1]4"/1
  Constant10/1 -> Divide3/1
  Sum5/1 -> Gain1/1
  Gain1/1 -> Divide3/2
  "[0,1]3"/1 -> [max_thigh_scale]
  Divide3/1 -> "[0,1]3"/1
  Constant9/1 -> Divide2/1
  Sum6/1 -> Divide2/2
  "[0,1]2"/1 -> [min_thigh_scale]
  Divide2/1 -> "[0,1]2"/1
  Gain/1 -> Divide1/2
  Constant8/1 -> Divide1/1
  Sum3/1 -> Gain/1
  "[0,1]1"/1 -> [max_splay_scale]
  Divide1/1 -> "[0,1]1"/1
  "[0,1]"/1 -> [min_splay_scale]
  Divide/1 -> "[0,1]"/1
  Sum4/1 -> Divide/2
  Constant7/1 -> Divide/1
  Constant/1 -> Sum/1
  Sum/1 -> scale_hip/1, Mux3/1
  [max_splay_scale] -> Mux7/2  "max_splay_scale"
  [min_splay_scale] -> Mux7/1  "min_splay_scale"
  Mux7/1 -> R scale hip/knee/3
  Mux8/1 -> R scale hip/knee/2
  [max_shin_scale] -> Mux8/2  "max_shin_scale"
  [min_shin_scale] -> Mux8/1  "min_shin_scale"
  Mux/1 -> R scale hip/knee/1
  [max_thigh_scale] -> Mux/2  "max_thigh_scale"
  [min_thigh_scale] -> Mux/1  "min_thigh_scale"
  Constant5/1 -> Sum7/1
  [shin] -> Sum7/2
  Constant6/1 -> Sum8/1
  [shin] -> Sum8/2
  Constant2/1 -> Sum5/1
  [thigh] -> Sum5/2
  Constant4/1 -> Sum6/1
  [thigh] -> Sum6/2
  Constant1/1 -> Sum3/1
  [splay] -> Sum3/2
  Constant3/1 -> Sum4/1
  [splay] -> Sum4/2
  Sum2/1 -> [splay]  "splay angle"
  phi_thigh [rad]/1 -> Sum2/2, [thigh]
  phi_shin [rad]/1 -> Sum2/1, [shin]

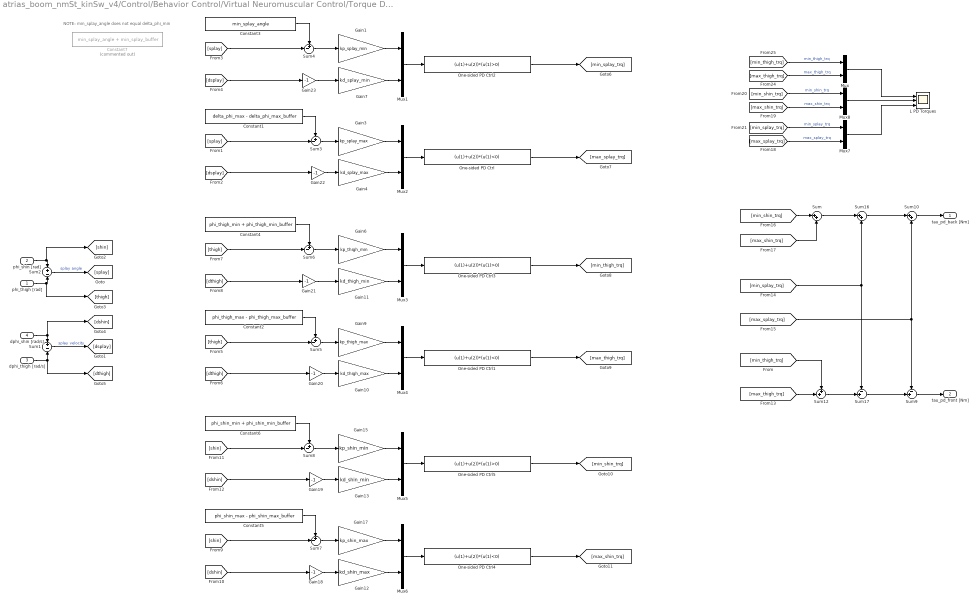
== system atrias_boom_nmSt_kinSw_v4/Control/Behavior Control/Virtual Neuromuscular Control/Torque Distribution/mech limit avoidance1/PD Joint Limit1/Lechanical Limit Avoidance Torques ==
  note: NOTE: min_splay_angle does not equal delta_phi_min
  phi_thigh [rad] : Inport
  phi_shin [rad] : Inport  Port=2
  dphi_thigh [rad/s] : Inport  Port=3
  dphi_shin [rad/s] : Inport  Port=4
  Constant1 : Constant  Value=delta_phi_max - delta_phi_max_buffer
  Constant2 : Constant  Value=phi_thigh_max - phi_thigh_max_buffer
  Constant3 : Constant  Value=min_splay_angle
  Constant4 : Constant  Value=phi_thigh_min + phi_thigh_min_buffer
  Constant5 : Constant  Value=phi_shin_max - phi_shin_max_buffer
  Constant6 : Constant  Value=phi_shin_min + phi_shin_min_buffer
  Constant7 : Constant  Commented=on  Value=min_splay_angle + min_splay_buffer
  Gain1 : Gain  Gain=kp_splay_min
  Gain10 : Gain  Gain=kd_thigh_max
  Gain11 : Gain  Gain=kd_thigh_min
  Gain12 : Gain  Gain=kd_shin_max
  Gain13 : Gain  Gain=kd_shin_min
  Gain15 : Gain  Gain=kp_shin_min
  Gain17 : Gain  Gain=kp_shin_max
  Gain{18..23} (6 alike) : Gain  Gain=-1
  Gain3 : Gain  Gain=kp_splay_max
  Gain4 : Gain  Gain=kd_splay_max
  Gain6 : Gain  Gain=kp_thigh_min
  Gain7 : Gain  Gain=kd_splay_min
  Gain9 : Gain  Gain=kp_thigh_max
  L PD Torques : Scope  NumInputPorts=3
      settings: ShowLegends=on  TimeRange=2.5  YMin=-100~-50000000~-10000000  YMax=100~10000000~50000000  SaveName=ScopeData5
  Mux{,1..8} (9 alike) : Mux  Inputs=2
  One-sided PD Ctrl : Fcn  Expr=(u(1)+u(2))*(u(1)<0)
  One-sided PD Ctrl1 : Fcn  Expr=(u(1)+u(2))*(u(1)<0)
  One-sided PD Ctrl2 : Fcn  Expr=(u(1)+u(2))*(u(1)>0)
  One-sided PD Ctrl3 : Fcn  Expr=(u(1)+u(2))*(u(1)>0)
  One-sided PD Ctrl4 : Fcn  Expr=(u(1)+u(2))*(u(1)<0)
  One-sided PD Ctrl5 : Fcn  Expr=(u(1)+u(2))*(u(1)>0)
  Sum : Sum  Inputs=|++
  Sum1 : Sum  Inputs=+-
  Sum10 : Sum  Inputs=|++
  Sum12 : Sum  Inputs=++|
  Sum16 : Sum  Inputs=|++
  Sum17 : Sum  Inputs=-+|
  Sum2 : Sum  Inputs=+-
  Sum{3..8} (6 alike) : Sum  Inputs=+-|
  Sum9 : Sum  Inputs=-+|
  tau_pd_back [Nm] : Outport
  tau_pd_front [Nm] : Outport  Port=2
  wires:
  dphi_shin [rad/s]/1 -> [dshin], Sum1/1
  dphi_thigh [rad/s]/1 -> [dthigh], Sum1/2
  phi_shin [rad]/1 -> [shin], Sum2/1
  phi_thigh [rad]/1 -> [thigh], Sum2/2
  Sum2/1 -> [splay]  "splay angle"
  Sum1/1 -> [dsplay]  "splay velocity"
  [dsplay] -> Gain23/1
  [splay] -> Sum4/2
  Gain7/1 -> Mux1/2
  Gain1/1 -> Mux1/1
  Sum4/1 -> Gain1/1
  Constant3/1 -> Sum4/1
  Mux1/1 -> One-sided PD Ctrl2/1
  [dsplay] -> Gain22/1
  [splay] -> Sum3/2
  Gain4/1 -> Mux2/2
  Gain3/1 -> Mux2/1
  Sum3/1 -> Gain3/1
  Constant1/1 -> Sum3/1
  Mux2/1 -> One-sided PD Ctrl/1
  [dthigh] -> Gain21/1
  [thigh] -> Sum6/2
  Gain11/1 -> Mux3/2
  Gain6/1 -> Mux3/1
  Sum6/1 -> Gain6/1
  Constant4/1 -> Sum6/1
  Mux3/1 -> One-sided PD Ctrl3/1
  [dthigh] -> Gain20/1
  [thigh] -> Sum5/2
  Gain10/1 -> Mux4/2
  Gain9/1 -> Mux4/1
  Sum5/1 -> Gain9/1
  Constant2/1 -> Sum5/1
  Mux4/1 -> One-sided PD Ctrl1/1
  [dshin] -> Gain19/1
  [shin] -> Sum8/2
  Gain13/1 -> Mux5/2
  Gain15/1 -> Mux5/1
  Sum8/1 -> Gain15/1
  Constant6/1 -> Sum8/1
  Mux5/1 -> One-sided PD Ctrl5/1
  [dshin] -> Gain18/1
  [shin] -> Sum7/2
  Gain12/1 -> Mux6/2
  Gain17/1 -> Mux6/1
  Sum7/1 -> Gain17/1
  Constant5/1 -> Sum7/1
  Mux6/1 -> One-sided PD Ctrl4/1
  One-sided PD Ctrl2/1 -> [min_splay_trq]
  [min_thigh_trq] -> Mux/1  "min_thigh_trq"
  [max_thigh_trq] -> Mux/2  "max_thigh_trq"
  Mux/1 -> L PD Torques/1
  [min_shin_trq] -> Mux8/1  "min_shin_trq"
  [max_shin_trq] -> Mux8/2  "max_shin_trq"
  Mux8/1 -> L PD Torques/2
  Mux7/1 -> L PD Torques/3
  [min_splay_trq] -> Mux7/1  "min_splay_trq"
  [max_splay_trq] -> Mux7/2  "max_splay_trq"
  Sum10/1 -> tau_pd_back [Nm]/1
  Sum9/1 -> tau_pd_front [Nm]/1
  Sum/1 -> Sum16/1
  [min_shin_trq] -> Sum/1
  [max_shin_trq] -> Sum/2
  Sum16/1 -> Sum10/1
  [min_splay_trq] -> Sum17/1, Sum16/2
  [max_splay_trq] -> Sum9/1, Sum10/2
  [max_thigh_trq] -> Sum12/2
  [min_thigh_trq] -> Sum12/1
  Sum12/1 -> Sum17/2
  Sum17/1 -> Sum9/2
  Gain18/1 -> Gain12/1
  Gain19/1 -> Gain13/1
  Gain20/1 -> Gain10/1
  Gain21/1 -> Gain11/1
  Gain22/1 -> Gain4/1
  Gain23/1 -> Gain7/1
  One-sided PD Ctrl/1 -> [max_splay_trq]
  One-sided PD Ctrl3/1 -> [min_thigh_trq]
  One-sided PD Ctrl1/1 -> [max_thigh_trq]
  One-sided PD Ctrl5/1 -> [min_shin_trq]
  One-sided PD Ctrl4/1 -> [max_shin_trq]

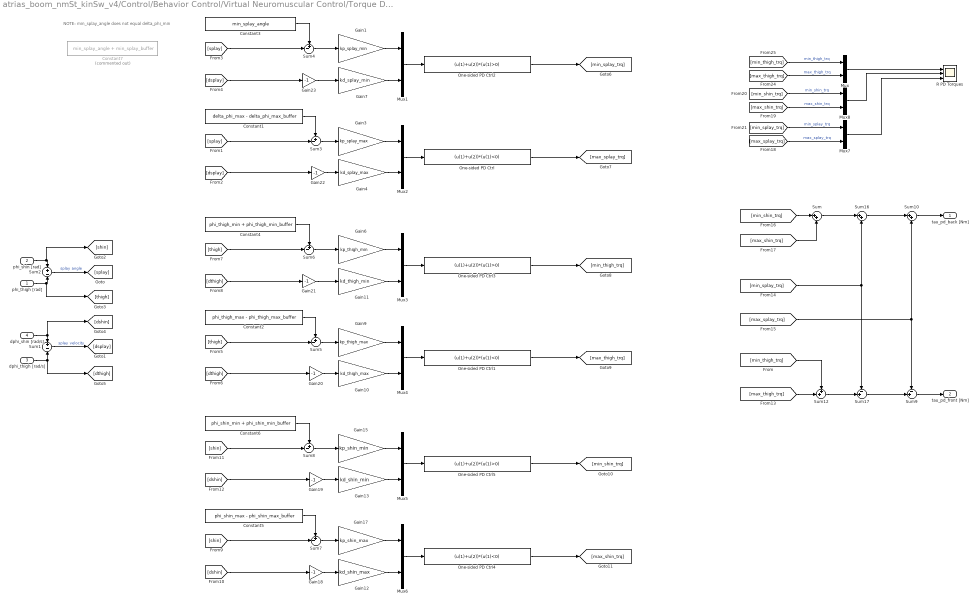
== system atrias_boom_nmSt_kinSw_v4/Control/Behavior Control/Virtual Neuromuscular Control/Torque Distribution/mech limit avoidance1/PD Joint Limit1/R Mechanical Limit Avoidance Torque ==
  note: NOTE: min_splay_angle does not equal delta_phi_min
  phi_thigh [rad] : Inport
  phi_shin [rad] : Inport  Port=2
  dphi_thigh [rad/s] : Inport  Port=3
  dphi_shin [rad/s] : Inport  Port=4
  Constant1 : Constant  Value=delta_phi_max - delta_phi_max_buffer
  Constant2 : Constant  Value=phi_thigh_max - phi_thigh_max_buffer
  Constant3 : Constant  Value=min_splay_angle
  Constant4 : Constant  Value=phi_thigh_min + phi_thigh_min_buffer
  Constant5 : Constant  Value=phi_shin_max - phi_shin_max_buffer
  Constant6 : Constant  Value=phi_shin_min + phi_shin_min_buffer
  Constant7 : Constant  Commented=on  Value=min_splay_angle + min_splay_buffer
  Gain1 : Gain  Gain=kp_splay_min
  Gain10 : Gain  Gain=kd_thigh_max
  Gain11 : Gain  Gain=kd_thigh_min
  Gain12 : Gain  Gain=kd_shin_max
  Gain13 : Gain  Gain=kd_shin_min
  Gain15 : Gain  Gain=kp_shin_min
  Gain17 : Gain  Gain=kp_shin_max
  Gain{18..23} (6 alike) : Gain  Gain=-1
  Gain3 : Gain  Gain=kp_splay_max
  Gain4 : Gain  Gain=kd_splay_max
  Gain6 : Gain  Gain=kp_thigh_min
  Gain7 : Gain  Gain=kd_splay_min
  Gain9 : Gain  Gain=kp_thigh_max
  Mux{,1..8} (9 alike) : Mux  Inputs=2
  One-sided PD Ctrl : Fcn  Expr=(u(1)+u(2))*(u(1)<0)
  One-sided PD Ctrl1 : Fcn  Expr=(u(1)+u(2))*(u(1)<0)
  One-sided PD Ctrl2 : Fcn  Expr=(u(1)+u(2))*(u(1)>0)
  One-sided PD Ctrl3 : Fcn  Expr=(u(1)+u(2))*(u(1)>0)
  One-sided PD Ctrl4 : Fcn  Expr=(u(1)+u(2))*(u(1)<0)
  One-sided PD Ctrl5 : Fcn  Expr=(u(1)+u(2))*(u(1)>0)
  R PD Torques : Scope  NumInputPorts=3
      settings: ShowLegends=on  TimeRange=2.5  YMin=-100~-50000000~-10000000  YMax=100~10000000~50000000  SaveName=ScopeData5
  Sum : Sum  Inputs=|++
  Sum1 : Sum  Inputs=+-
  Sum10 : Sum  Inputs=|++
  Sum12 : Sum  Inputs=++|
  Sum16 : Sum  Inputs=|++
  Sum17 : Sum  Inputs=-+|
  Sum2 : Sum  Inputs=+-
  Sum{3..8} (6 alike) : Sum  Inputs=+-|
  Sum9 : Sum  Inputs=-+|
  tau_pd_back [Nm] : Outport
  tau_pd_front [Nm] : Outport  Port=2
  wires:
  One-sided PD Ctrl4/1 -> [max_shin_trq]
  One-sided PD Ctrl5/1 -> [min_shin_trq]
  One-sided PD Ctrl1/1 -> [max_thigh_trq]
  One-sided PD Ctrl3/1 -> [min_thigh_trq]
  One-sided PD Ctrl/1 -> [max_splay_trq]
  Gain23/1 -> Gain7/1
  Gain22/1 -> Gain4/1
  Gain21/1 -> Gain11/1
  Gain20/1 -> Gain10/1
  Gain19/1 -> Gain13/1
  Gain18/1 -> Gain12/1
  Sum17/1 -> Sum9/2
  Sum12/1 -> Sum17/2
  [min_thigh_trq] -> Sum12/1
  [max_thigh_trq] -> Sum12/2
  [max_splay_trq] -> Sum10/2, Sum9/1
  [min_splay_trq] -> Sum16/2, Sum17/1
  Sum16/1 -> Sum10/1
  [max_shin_trq] -> Sum/2
  [min_shin_trq] -> Sum/1
  Sum/1 -> Sum16/1
  Sum9/1 -> tau_pd_front [Nm]/1
  Sum10/1 -> tau_pd_back [Nm]/1
  [max_splay_trq] -> Mux7/2  "max_splay_trq"
  [min_splay_trq] -> Mux7/1  "min_splay_trq"
  Mux7/1 -> R PD Torques/3
  Mux8/1 -> R PD Torques/2
  [max_shin_trq] -> Mux8/2  "max_shin_trq"
  [min_shin_trq] -> Mux8/1  "min_shin_trq"
  Mux/1 -> R PD Torques/1
  [max_thigh_trq] -> Mux/2  "max_thigh_trq"
  [min_thigh_trq] -> Mux/1  "min_thigh_trq"
  One-sided PD Ctrl2/1 -> [min_splay_trq]
  Mux6/1 -> One-sided PD Ctrl4/1
  Constant5/1 -> Sum7/1
  Sum7/1 -> Gain17/1
  Gain17/1 -> Mux6/1
  Gain12/1 -> Mux6/2
  [shin] -> Sum7/2
  [dshin] -> Gain18/1
  Mux5/1 -> One-sided PD Ctrl5/1
  Constant6/1 -> Sum8/1
  Sum8/1 -> Gain15/1
  Gain15/1 -> Mux5/1
  Gain13/1 -> Mux5/2
  [shin] -> Sum8/2
  [dshin] -> Gain19/1
  Mux4/1 -> One-sided PD Ctrl1/1
  Constant2/1 -> Sum5/1
  Sum5/1 -> Gain9/1
  Gain9/1 -> Mux4/1
  Gain10/1 -> Mux4/2
  [thigh] -> Sum5/2
  [dthigh] -> Gain20/1
  Mux3/1 -> One-sided PD Ctrl3/1
  Constant4/1 -> Sum6/1
  Sum6/1 -> Gain6/1
  Gain6/1 -> Mux3/1
  Gain11/1 -> Mux3/2
  [thigh] -> Sum6/2
  [dthigh] -> Gain21/1
  Mux2/1 -> One-sided PD Ctrl/1
  Constant1/1 -> Sum3/1
  Sum3/1 -> Gain3/1
  Gain3/1 -> Mux2/1
  Gain4/1 -> Mux2/2
  [splay] -> Sum3/2
  [dsplay] -> Gain22/1
  Mux1/1 -> One-sided PD Ctrl2/1
  Constant3/1 -> Sum4/1
  Sum4/1 -> Gain1/1
  Gain1/1 -> Mux1/1
  Gain7/1 -> Mux1/2
  [splay] -> Sum4/2
  [dsplay] -> Gain23/1
  Sum1/1 -> [dsplay]  "splay velocity"
  Sum2/1 -> [splay]  "splay angle"
  phi_thigh [rad]/1 -> Sum2/2, [thigh]
  phi_shin [rad]/1 -> Sum2/1, [shin]
  dphi_thigh [rad/s]/1 -> Sum1/2, [dthigh]
  dphi_shin [rad/s]/1 -> Sum1/1, [dshin]

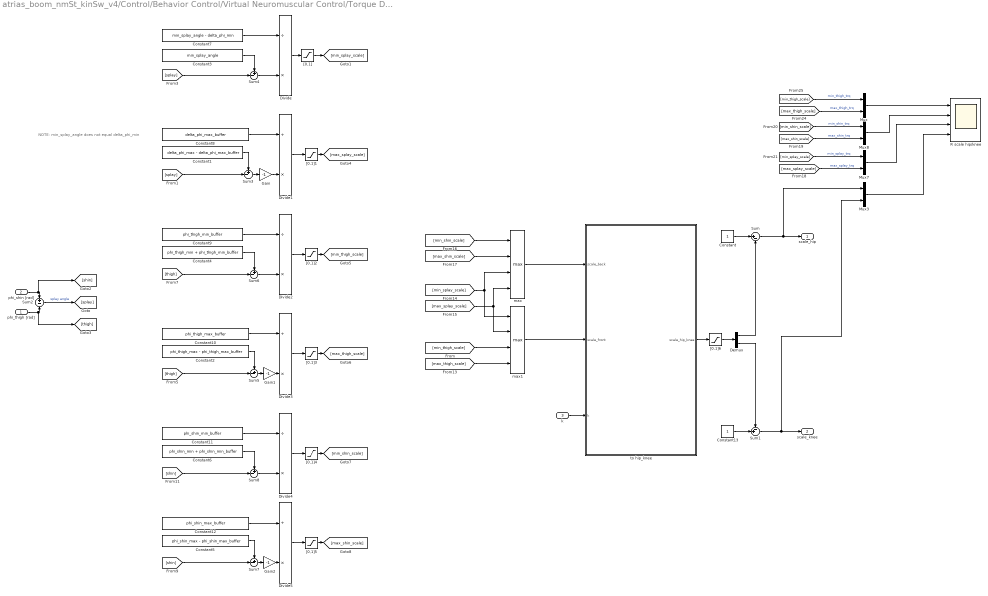
== system atrias_boom_nmSt_kinSw_v4/Control/Behavior Control/Virtual Neuromuscular Control/Torque Distribution/mech limit avoidance1/PD Joint Limit1/R scale desired torque ==
  note: NOTE: min_splay_angle does not equal delta_phi_min
  phi_thigh [rad] : Inport
  phi_shin [rad] : Inport  Port=2
  k : Inport  Port=3
  Constant : Constant
  Constant1 : Constant  Value=delta_phi_max - delta_phi_max_buffer
  Constant10 : Constant  Value=phi_thigh_max_buffer
  Constant11 : Constant  Value=phi_shin_min_buffer
  Constant12 : Constant  Value=phi_shin_max_buffer
  Constant13 : Constant
  Constant2 : Constant  Value=phi_thigh_max - phi_thigh_max_buffer
  Constant3 : Constant  Value=min_splay_angle
  Constant4 : Constant  Value=phi_thigh_min + phi_thigh_min_buffer
  Constant5 : Constant  Value=phi_shin_max - phi_shin_max_buffer
  Constant6 : Constant  Value=phi_shin_min + phi_shin_min_buffer
  Constant7 : Constant  Value=min_splay_angle - delta_phi_min
  Constant8 : Constant  Value=delta_phi_max_buffer
  Constant9 : Constant  Value=phi_thigh_min_buffer
  Demux : Demux  Outputs=2
  Divide{,1..5} (6 alike) : Product  Inputs=/*
  Gain : Gain  Gain=-1
  Gain1 : Gain  Gain=-1
  Gain2 : Gain  Gain=-1
  Mux{,3,7..8} (4 alike) : Mux  Inputs=2
  R scale hip/knee : Scope  NumInputPorts=4
      settings: ShowLegends=on  TimeRange=2.5  YMin=-100~-5e+07~-1e+07~-5  YMax=100~1e+07~5e+07~5  SaveName=ScopeData5
  Sum : Sum  Inputs=|+-
  Sum1 : Sum  Inputs=-+|
  Sum2 : Sum  Inputs=+-
  Sum{3..8} (6 alike) : Sum  Inputs=+-|
  [0,1]{,1..6} (7 alike) : Saturate  UpperLimit=1  LowerLimit=0
  max : MinMax  Function=max  Inputs=4
  max1 : MinMax  Function=max  Inputs=4
  to hip_knee : MATLAB Function  TreatAsAtomicUnit=on
  scale_hip : Outport
  scale_knee : Outport  Port=2
  wires:
  phi_shin [rad]/1 -> [shin], Sum2/1
  phi_thigh [rad]/1 -> [thigh], Sum2/2
  Sum2/1 -> [splay]  "splay angle"
  [splay] -> Sum4/2
  Constant3/1 -> Sum4/1
  [splay] -> Sum3/2
  Constant1/1 -> Sum3/1
  [thigh] -> Sum6/2
  Constant4/1 -> Sum6/1
  [thigh] -> Sum5/2
  Constant2/1 -> Sum5/1
  [shin] -> Sum8/2
  Constant6/1 -> Sum8/1
  [shin] -> Sum7/2
  Constant5/1 -> Sum7/1
  [min_thigh_scale] -> Mux/1  "min_thigh_trq"
  [max_thigh_scale] -> Mux/2  "max_thigh_trq"
  Mux/1 -> R scale hip/knee/1
  [min_shin_scale] -> Mux8/1  "min_shin_trq"
  [max_shin_scale] -> Mux8/2  "max_shin_trq"
  Mux8/1 -> R scale hip/knee/2
  Mux7/1 -> R scale hip/knee/3
  [min_splay_scale] -> Mux7/1  "min_splay_trq"
  [max_splay_scale] -> Mux7/2  "max_splay_trq"
  Sum/1 -> Mux3/1, scale_hip/1
  Constant/1 -> Sum/1
  Constant7/1 -> Divide/1
  Sum4/1 -> Divide/2
  Divide/1 -> "[0,1]"/1
  "[0,1]"/1 -> [min_splay_scale]
  Divide1/1 -> "[0,1]1"/1
  "[0,1]1"/1 -> [max_splay_scale]
  Sum3/1 -> Gain/1
  Constant8/1 -> Divide1/1
  Gain/1 -> Divide1/2
  Divide2/1 -> "[0,1]2"/1
  "[0,1]2"/1 -> [min_thigh_scale]
  Sum6/1 -> Divide2/2
  Constant9/1 -> Divide2/1
  Divide3/1 -> "[0,1]3"/1
  "[0,1]3"/1 -> [max_thigh_scale]
  Gain1/1 -> Divide3/2
  Sum5/1 -> Gain1/1
  Constant10/1 -> Divide3/1
  Divide4/1 -> "[0,1]4"/1
  "[0,1]4"/1 -> [min_shin_scale]
  Sum8/1 -> Divide4/2
  Constant11/1 -> Divide4/1
  Divide5/1 -> "[0,1]5"/1
  "[0,1]5"/1 -> [max_shin_scale]
  Sum7/1 -> Gain2/1
  Constant12/1 -> Divide5/1
  Gain2/1 -> Divide5/2
  Constant13/1 -> Sum1/2
  [min_shin_scale] -> max/1
  [max_shin_scale] -> max/2
  [min_splay_scale] -> max1/1, max/3
  [max_splay_scale] -> max1/2, max/4
  [max_thigh_scale] -> max1/4
  [min_thigh_scale] -> max1/3
  Sum1/1 -> Mux3/2, scale_knee/1
  max/1 -> to hip_knee/1(scale_back)
  max1/1 -> to hip_knee/2(scale_front)
  k/1 -> to hip_knee/3(k)
  to hip_knee/1(scale_hip_knee) -> "[0,1]6"/1
  Demux/1 -> Sum/2
  Demux/2 -> Sum1/1
  Mux3/1 -> R scale hip/knee/4
  "[0,1]6"/1 -> Demux/1
